simulink model "LyapunovController"  (R2022b)
settings: Solver=VariableStepAuto  StartTime=0.0  StopTime=50  RelTol=1e-3
model workspace (MAT data in the model file):
  Sig = Simulink.Signal
  Sig.DataType = 'auto'
  Sig.Dimensions = -1
  Sig.DimensionsMode = 'auto'
  Sig.Complexity = 'auto'
  Sig.SampleTime = -1
  Sig.SamplingMode = 'auto'
values from neighbouring files (symbols this model uses):
  Kt = 10    [Lyapunov.m]
  Kx = 5    [Lyapunov.m]
  thetad = 180    [Lyapunov.m]
  xd = 200    [Lyapunov.m]
  yd = 100    [Lyapunov.m]
libraries: simulink_extras x5
settings Model: Creator=The MathWorks, Inc.  LastModifiedBy=MuAyman
settings SolverCC: AlgebraicLoopSolver=TrustRegion
settings DebuggingCC: UnconnectedInputMsg=warning  UnconnectedOutputMsg=warning  UnconnectedLineMsg=warning  SymbolicDimsDataTypeCodeGenerationDiagnostic=none  SFMachineParentedDataDiag=warning
settings ModelReferenceCC: EnableRefExpFcnMdlSchedulingChecks=on
settings RTWCC: DLArmComputeVersion=19.05

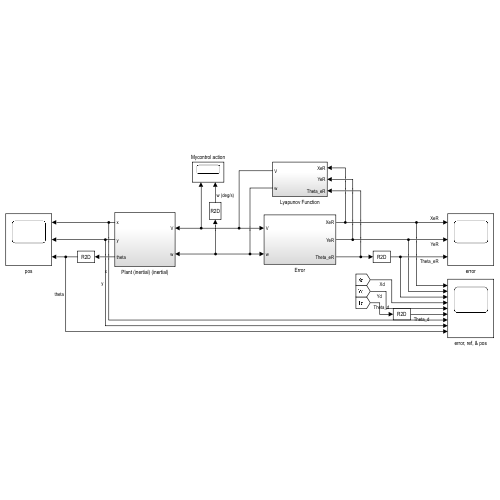
[thumbnail: Simulink's stored preview of the top-level diagram]
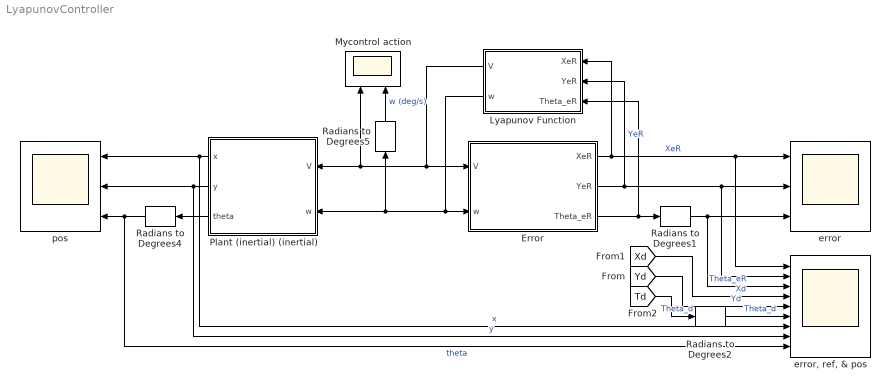
== system LyapunovController ==
  Error : Subsystem
  Lyapunov Function : Subsystem
  Mycontrol action : Scope  NumInputPorts=2
  Plant (inertial) (inertial) : Subsystem
  Radians to Degrees{1..2,4..5} (4 alike) : simulink_extras/Transformations/Radians to Degrees
  error : Scope  NumInputPorts=3
  "error, ref, & pos" : Scope  NumInputPorts=9
  pos : Scope  NumInputPorts=3
  wires:
  Radians to Degrees5/1 -> Mycontrol action/2  "w (deg/s)"
  Error/2(YeR) -> "error, ref, & pos"/2, error/2, Lyapunov Function/2(YeR)  "YeR"
  Error/3(Theta_eR) -> Lyapunov Function/3(Theta_eR), Radians to Degrees1/1
  Error/1(XeR) -> error/1, "error, ref, & pos"/1, Lyapunov Function/1(XeR)  "XeR"
  Radians to Degrees1/1 -> "error, ref, & pos"/3, error/3  "Theta_eR"
  [Xd] -> "error, ref, & pos"/4  "Xd"
  [Yd] -> "error, ref, & pos"/5  "Yd"
  [Td] -> Radians to Degrees2/1  "Theta_d"
  Lyapunov Function/2(w) -> Plant (inertial) (inertial)/2(w), Radians to Degrees5/1, Error/2(w)
  Plant (inertial) (inertial)/3(theta) -> Radians to Degrees4/1
  Lyapunov Function/1(V) -> Plant (inertial) (inertial)/1(V), Mycontrol action/1, Error/1(V)
  Radians to Degrees4/1 -> pos/3, "error, ref, & pos"/9  "theta"
  Plant (inertial) (inertial)/2(y) -> pos/2, "error, ref, & pos"/8  "y"
  Plant (inertial) (inertial)/1(x) -> pos/1, "error, ref, & pos"/7  "x"
  Radians to Degrees2/1 -> "error, ref, & pos"/6  "Theta_d"

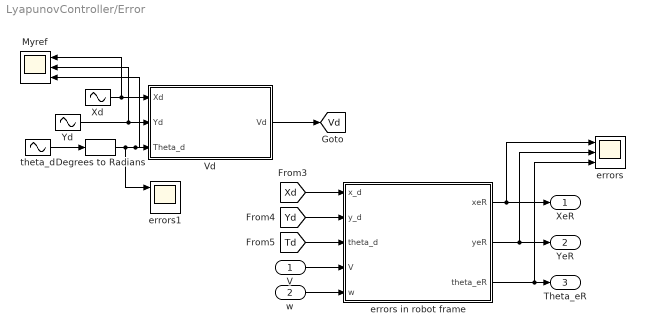
== system LyapunovController/Error ==
  V : Inport
  w : Inport  Port=2
  Degrees to Radians : simulink_extras/Transformations/Degrees to Radians
  Myref : Scope  NumInputPorts=3
  Vd : Subsystem
  Xd : Sin  Amplitude=xd  Phase=pi/4  SampleTime=0
  Yd : Sin  Amplitude=yd  Phase=pi/4  SampleTime=0
  errors : Scope  NumInputPorts=3
  errors in robot frame : Subsystem
  errors1 : Scope  NumInputPorts=3
  theta_d : Sin  Amplitude=thetad  Phase=pi/4  SampleTime=0
  XeR : Outport
  YeR : Outport  Port=2
  Theta_eR : Outport  Port=3
  tag scope: Vd=global
  wires:
  w/1 -> errors in robot frame/5(w)
  V/1 -> errors in robot frame/4(V)
  Vd/1(Vd) -> [Vd]
  Xd/1 -> Myref/1, Vd/1(Xd)
  Yd/1 -> Myref/2, Vd/2(Yd)
  theta_d/1 -> Degrees to Radians/1
  errors in robot frame/2(yeR) -> YeR/1, errors/2
  errors in robot frame/3(theta_eR) -> errors/3, Theta_eR/1
  errors in robot frame/1(xeR) -> XeR/1, errors/1
  [Yd] -> errors in robot frame/2(y_d)
  [Xd] -> errors in robot frame/1(x_d)
  [Td] -> errors in robot frame/3(theta_d)
  Degrees to Radians/1 -> errors1/1, Myref/3, Vd/3(Theta_d)

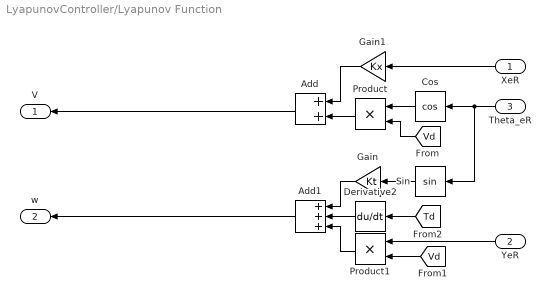
== system LyapunovController/Lyapunov Function ==
  XeR : Inport
  YeR : Inport  Port=2
  Theta_eR : Inport  Port=3
  Add : Sum
  Add1 : Sum  Inputs=+++
  Cos : Trigonometry  Operator=cos
  Derivative2 : Derivative
  Gain : Gain  Gain=Kt
  Gain1 : Gain  Gain=Kx
  Product : Product
  Product1 : Product
  Sin : Trigonometry
  V : Outport
  w : Outport  Port=2
  wires:
  [Vd] -> Product1/2
  [Vd] -> Product/2
  Product/1 -> Add/2
  Sin/1 -> Gain/1
  [Td] -> Derivative2/1
  Cos/1 -> Product/1
  Gain1/1 -> Add/1
  Gain/1 -> Add1/1
  Product1/1 -> Add1/3
  XeR/1 -> Gain1/1
  Theta_eR/1 -> Sin/1, Cos/1
  Add1/1 -> w/1
  YeR/1 -> Product1/1
  Add/1 -> V/1
  Derivative2/1 -> Add1/2

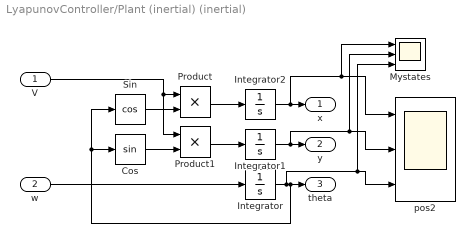
== system LyapunovController/Plant (inertial) (inertial) ==
  V : Inport
  w : Inport  Port=2
  Cos : Trigonometry
  Integrator : Integrator
  Integrator1 : Integrator
  Integrator2 : Integrator
  Mystates : Scope  NumInputPorts=3
  Product : Product
  Product1 : Product
  Sin : Trigonometry  Operator=cos
  pos2 : Scope  NumInputPorts=3
  x : Outport
  y : Outport  Port=2
  theta : Outport  Port=3
  wires:
  Integrator/1 -> pos2/3, Mystates/3, Cos/1, Sin/1, theta/1
  w/1 -> Integrator/1
  Sin/1 -> Product/2
  Cos/1 -> Product1/2
  Product1/1 -> Integrator1/1
  Product/1 -> Integrator2/1
  Integrator1/1 -> Mystates/2, pos2/2, y/1
  Integrator2/1 -> Mystates/1, pos2/1, x/1
  V/1 -> Product1/1, Product/1

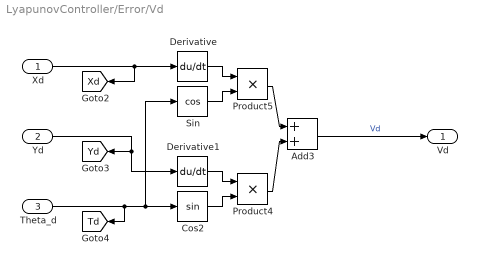
== system LyapunovController/Error/Vd ==
  Xd : Inport
  Yd : Inport  Port=2
  Theta_d : Inport  Port=3
  Add3 : Sum
  Cos2 : Trigonometry
  Derivative : Derivative
  Derivative1 : Derivative
  Product4 : Product
  Product5 : Product
  Sin : Trigonometry  Operator=cos
  Vd : Outport
  tag scope: Td=global, Xd=global, Yd=global
  wires:
  Theta_d/1 -> [Td], Sin/1, Cos2/1
  Sin/1 -> Product5/2
  Derivative/1 -> Product5/1
  Product5/1 -> Add3/1
  Product4/1 -> Add3/2
  Cos2/1 -> Product4/2
  Derivative1/1 -> Product4/1
  Add3/1 -> Vd/1  "Vd"
  Yd/1 -> [Yd], Derivative1/1
  Xd/1 -> [Xd], Derivative/1

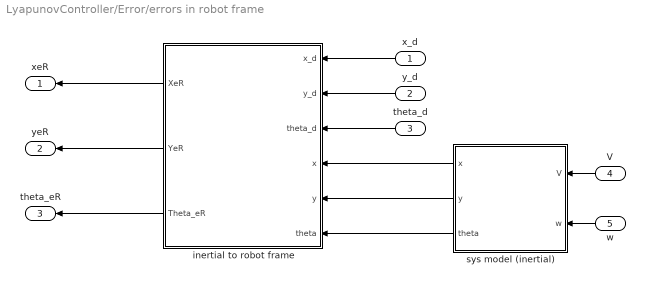
== system LyapunovController/Error/errors in robot frame ==
  x_d : Inport
  y_d : Inport  Port=2
  theta_d : Inport  Port=3
  V : Inport  Port=4
  w : Inport  Port=5
  inertial to robot frame : Subsystem
  sys model (inertial) : Subsystem
  xeR : Outport
  yeR : Outport  Port=2
  theta_eR : Outport  Port=3
  wires:
  w/1 -> sys model (inertial)/2(w)
  V/1 -> sys model (inertial)/1(V)
  x_d/1 -> inertial to robot frame/1(x_d)
  y_d/1 -> inertial to robot frame/2(y_d)
  theta_d/1 -> inertial to robot frame/3(theta_d)
  sys model (inertial)/1(x) -> inertial to robot frame/4(x)
  sys model (inertial)/2(y) -> inertial to robot frame/5(y)
  sys model (inertial)/3(theta) -> inertial to robot frame/6(theta)
  inertial to robot frame/1(XeR) -> xeR/1
  inertial to robot frame/2(YeR) -> yeR/1
  inertial to robot frame/3(Theta_eR) -> theta_eR/1

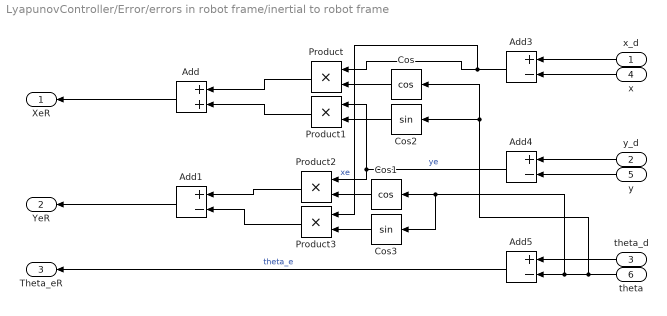
== system LyapunovController/Error/errors in robot frame/inertial to robot frame ==
  x_d : Inport
  y_d : Inport  Port=2
  theta_d : Inport  Port=3
  x : Inport  Port=4
  y : Inport  Port=5
  theta : Inport  Port=6
  Add : Sum
  Add{1,3..5} (4 alike) : Sum  Inputs=+-
  Cos : Trigonometry  Operator=cos
  Cos1 : Trigonometry  Operator=cos
  Cos2 : Trigonometry
  Cos3 : Trigonometry
  Product{,1..3} (4 alike) : Product
  XeR : Outport
  YeR : Outport  Port=2
  Theta_eR : Outport  Port=3
  wires:
  theta_d/1 -> Add5/1
  Add4/1 -> Product2/1, Product1/1  "ye"
  y_d/1 -> Add4/1
  Add5/1 -> Theta_eR/1  "theta_e"
  x/1 -> Add3/2
  x_d/1 -> Add3/1
  y/1 -> Add4/2
  theta/1 -> Cos2/1, Cos/1, Cos3/1, Cos1/1, Add5/2
  Cos/1 -> Product/2
  Add3/1 -> Product3/1, Product/1  "xe"
  Product/1 -> Add/1
  Cos2/1 -> Product1/2
  Product1/1 -> Add/2
  Add/1 -> XeR/1
  Cos1/1 -> Product2/2
  Cos3/1 -> Product3/2
  Product2/1 -> Add1/1
  Product3/1 -> Add1/2
  Add1/1 -> YeR/1

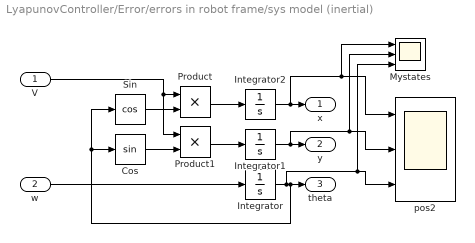
== system LyapunovController/Error/errors in robot frame/sys model (inertial) ==
  V : Inport
  w : Inport  Port=2
  Cos : Trigonometry
  Integrator : Integrator
  Integrator1 : Integrator
  Integrator2 : Integrator
  Mystates : Scope  NumInputPorts=3
  Product : Product
  Product1 : Product
  Sin : Trigonometry  Operator=cos
  pos2 : Scope  NumInputPorts=3
  x : Outport
  y : Outport  Port=2
  theta : Outport  Port=3
  wires:
  Integrator/1 -> pos2/3, Mystates/3, Cos/1, Sin/1, theta/1
  w/1 -> Integrator/1
  Sin/1 -> Product/2
  Cos/1 -> Product1/2
  Product1/1 -> Integrator1/1
  Product/1 -> Integrator2/1
  Integrator1/1 -> Mystates/2, pos2/2, y/1
  Integrator2/1 -> Mystates/1, pos2/1, x/1
  V/1 -> Product1/1, Product/1
